simulink model "simulink_example"  (R2016a)
settings: Solver=ode1  StartTime=0.0  StopTime=inf  FixedStep=0.001  RelTol=1e-3
undefined symbols (not defined in the file): serial
libraries: dspswit3 x2, instrumentlib x2
settings Model: Creator=Andrei  LastModifiedBy=Andrei

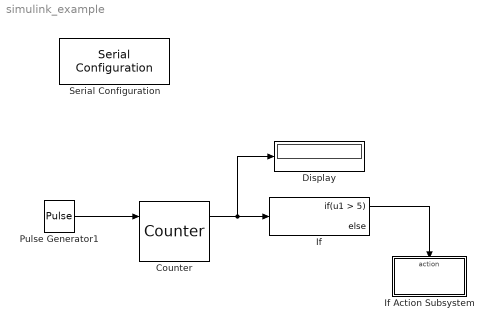
== system simulink_example ==
  Counter : dspswit3/Counter  Direction=Up  CountEvent=Falling edge  CounterSize=8 bits  MaxCount=255  InitialCount=0  Output=Count and Hit  HitValue=32  ResetInput=on  SamplesPerFrame=1  Ts=1  CntDtype=uint8  HitDtype=Logical
  Display : Display
  If : If  IfExpression=u1 > 5
  If Action Subsystem : Subsystem  TreatAsAtomicUnit=on
  Pulse Generator1 : DiscretePulseGenerator  PulseType=Time based  Period=100  PulseWidth=50
  Serial Configuration : instrumentlib/Serial Configuration  Priority=-200000  ComPortMenu=COM3  ComPort=COM3  ObjConstructor=serial('COM3');  BaudRate=9600  DataBits=8  Parity=none  StopBits=1  FlowControl=none  Timeout=10  ByteOrder=LittleEndian
  wires:
  If/1 -> If Action Subsystem/Action
  Counter/1 -> Display/1, If/1
  Pulse Generator1/1 -> Counter/1

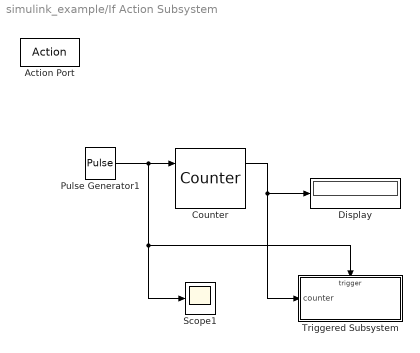
== system simulink_example/If Action Subsystem ==
  Action Port : ActionPort  ActionType=then
  Counter : dspswit3/Counter  Direction=Up  CountEvent=Falling edge  CounterSize=8 bits  MaxCount=255  InitialCount=0  Output=Count and Hit  HitValue=32  ResetInput=on  SamplesPerFrame=1  Ts=1  CntDtype=uint8  HitDtype=Logical
  Display : Display
  Pulse Generator1 : DiscretePulseGenerator  PulseType=Time based  Period=5  PulseWidth=50
  Scope1 : Scope
  Triggered Subsystem : Subsystem  TreatAsAtomicUnit=on
  wires:
  Pulse Generator1/1 -> Counter/1, Triggered Subsystem/Trigger, Scope1/1
  Counter/1 -> Triggered Subsystem/1(counter), Display/1

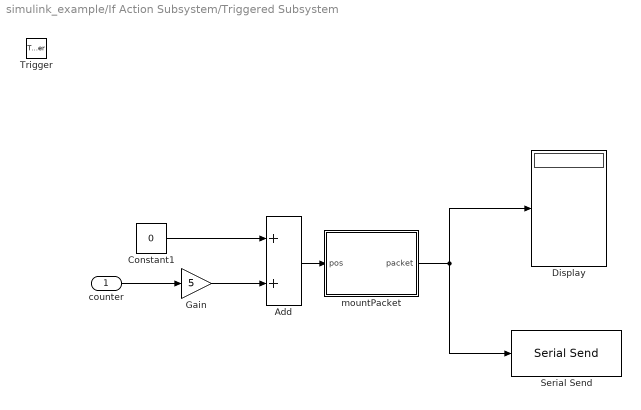
== system simulink_example/If Action Subsystem/Triggered Subsystem ==
  counter : Inport  OutDataTypeStr=uint8
  Trigger : TriggerPort  TriggerType=falling  VariantControl=Variant
  Add : Sum  OutDataTypeStr=uint16
  Constant1 : Constant  Value=0  OutDataTypeStr=uint8
  Display : Display
  Gain : Gain  Gain=5
  Serial Send : instrumentlib/Serial Send  ComPortMenu=COM3  ComPort=COM3  ObjConstructor=serial('COM3');  Terminator=<none>  EnableBlockingMode=on
  mountPacket : MATLAB Function  TreatAsAtomicUnit=on
  wires:
  counter/1 -> Gain/1
  Constant1/1 -> Add/1
  Add/1 -> mountPacket/1(pos)
  mountPacket/1(packet) -> Display/1, Serial Send/1
  Gain/1 -> Add/2

== matlab function simulink_example/If Action Subsystem/Triggered Subsystem/mountPacket ==
  data: pos input; packet output
function packet = sendSerialData(pos)
    posMSB = uint8(bitshift(pos,-8)); %equivalent to pos>>8
    posLSB = uint8(bitand(pos,255)); %equivalent to pos&0XFF
    packet = uint8(zeros(1,6));
    packet(1) = uint8(36); %header: '$'
    packet(2) = uint8(0); %action
    packet(3) = uint8(6); %servo
    packet(4) = uint8(posMSB); %posMSB
    packet(5) = uint8(posLSB); %posLSB
    packet(6) = uint8(33); %end package: '!'
    packet = uint8(packet);
end
